simulink model "simulink_test"  (R2018a)
settings: Solver=FixedStepAuto  StartTime=0.0  StopTime=5  FixedStep=1  RelTol=1e-3
undefined symbols (not defined in the file): init, stop
settings Model: Creator=root  LastModifiedBy=root

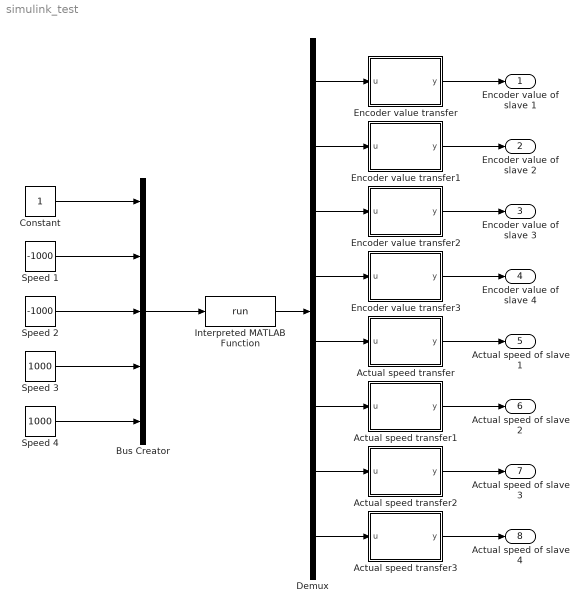
== system simulink_test ==
  Actual speed transfer : MATLAB Function  TreatAsAtomicUnit=on
  Actual speed transfer1 : MATLAB Function  TreatAsAtomicUnit=on
  Actual speed transfer2 : MATLAB Function  TreatAsAtomicUnit=on
  Actual speed transfer3 : MATLAB Function  TreatAsAtomicUnit=on
  Bus Creator : BusCreator  Inputs=5
  Constant : Constant
  Demux : Demux  Outputs=8
  Encoder value transfer : MATLAB Function  TreatAsAtomicUnit=on
  Encoder value transfer1 : MATLAB Function  TreatAsAtomicUnit=on
  Encoder value transfer2 : MATLAB Function  TreatAsAtomicUnit=on
  Encoder value transfer3 : MATLAB Function  TreatAsAtomicUnit=on
  Interpreted MATLAB Function : MATLABFcn  StartFcn=init([1])  StopFcn=stop([1])  MATLABFcn=run
  Speed 1 : Constant  Value=-1000
  Speed 2 : Constant  Value=-1000
  Speed 3 : Constant  Value=1000
  Speed 4 : Constant  Value=1000
  Encoder value of slave 1 : Outport
  Encoder value of slave 2 : Outport  Port=2
  Encoder value of slave 3 : Outport  Port=3
  Encoder value of slave 4 : Outport  Port=4
  Actual speed of slave 1 : Outport  Port=5
  Actual speed of slave 2 : Outport  Port=6
  Actual speed of slave 3 : Outport  Port=7
  Actual speed of slave 4 : Outport  Port=8
  wires:
  Constant/1 -> Bus Creator/1
  Bus Creator/1 -> Interpreted MATLAB Function/1
  Speed 1/1 -> Bus Creator/2
  Interpreted MATLAB Function/1 -> Demux/1
  Demux/1 -> Encoder value transfer/1(u)
  Encoder value transfer/1(y) -> Encoder value of slave 1/1
  Actual speed transfer/1(y) -> Actual speed of slave 1/1
  Demux/5 -> Actual speed transfer/1(u)
  Demux/4 -> Encoder value transfer3/1(u)
  Demux/3 -> Encoder value transfer2/1(u)
  Demux/2 -> Encoder value transfer1/1(u)
  Encoder value transfer1/1(y) -> Encoder value of slave 2/1
  Encoder value transfer2/1(y) -> Encoder value of slave 3/1
  Encoder value transfer3/1(y) -> Encoder value of slave 4/1
  Demux/6 -> Actual speed transfer1/1(u)
  Demux/7 -> Actual speed transfer2/1(u)
  Demux/8 -> Actual speed transfer3/1(u)
  Actual speed transfer1/1(y) -> Actual speed of slave 2/1
  Actual speed transfer2/1(y) -> Actual speed of slave 3/1
  Actual speed transfer3/1(y) -> Actual speed of slave 4/1
  Speed 2/1 -> Bus Creator/3
  Speed 3/1 -> Bus Creator/4
  Speed 4/1 -> Bus Creator/5

== matlab function simulink_test/Actual speed transfer ==
  data: u input; y output
function y = fcn(u)
if (u > 4000000000)
    a = dec2bin(u - 1, 32);
    k = 32;
    for k = 1:32
        if a(k) == '0'
            a(k) = '1';
        else
            a(k) = '0';
        end
    end
    y = bin2dec(a)*(-1);
else
    y = u;
end

== matlab function simulink_test/Encoder value transfer ==
  data: u input; y output
function y = fcn(u)
if (u > 4290000000)
    a = dec2bin(u - 1, 32);
    k = 32;
    for k = 1:32
        if a(k) == '0'
            a(k) = '1';
        else
            a(k) = '0';
        end
    end
    y = bin2dec(a)*(-1);
else
    y = u;
end

== matlab function simulink_test/Encoder value transfer1 ==
  data: u input; y output
function y = fcn(u)
if (u > 4290000000)
    a = dec2bin(u - 1, 32);
    k = 32;
    for k = 1:32
        if a(k) == '0'
            a(k) = '1';
        else
            a(k) = '0';
        end
    end
    y = bin2dec(a)*(-1);
else
    y = u;
end

== matlab function simulink_test/Encoder value transfer2 ==
  data: u input; y output
function y = fcn(u)
if (u > 4290000000)
    a = dec2bin(u - 1, 32);
    k = 32;
    for k = 1:32
        if a(k) == '0'
            a(k) = '1';
        else
            a(k) = '0';
        end
    end
    y = bin2dec(a)*(-1);
else
    y = u;
end

== matlab function simulink_test/Encoder value transfer3 ==
  data: u input; y output
function y = fcn(u)
if (u > 4290000000)
    a = dec2bin(u - 1, 32);
    k = 32;
    for k = 1:32
        if a(k) == '0'
            a(k) = '1';
        else
            a(k) = '0';
        end
    end
    y = bin2dec(a)*(-1);
else
    y = u;
end

== matlab function simulink_test/Actual speed transfer1 ==
  data: u input; y output
function y = fcn(u)
if (u > 4000000000)
    a = dec2bin(u - 1, 32);
    k = 32;
    for k = 1:32
        if a(k) == '0'
            a(k) = '1';
        else
            a(k) = '0';
        end
    end
    y = bin2dec(a)*(-1);
else
    y = u;
end

== matlab function simulink_test/Actual speed transfer2 ==
  data: u input; y output
function y = fcn(u)
if (u > 4000000000)
    a = dec2bin(u - 1, 32);
    k = 32;
    for k = 1:32
        if a(k) == '0'
            a(k) = '1';
        else
            a(k) = '0';
        end
    end
    y = bin2dec(a)*(-1);
else
    y = u;
end

== matlab function simulink_test/Actual speed transfer3 ==
  data: u input; y output
function y = fcn(u)
if (u > 4000000000)
    a = dec2bin(u - 1, 32);
    k = 32;
    for k = 1:32
        if a(k) == '0'
            a(k) = '1';
        else
            a(k) = '0';
        end
    end
    y = bin2dec(a)*(-1);
else
    y = u;
end
